simulink model "fullDiveHarness"  (R2026a)
settings: Solver=ode23t  StopTime=3900  MaxStep=0.1  RelTol=1e-4
libraries: simulink x2
settings Model: Creator=grouleau  LastModifiedBy=grouleau

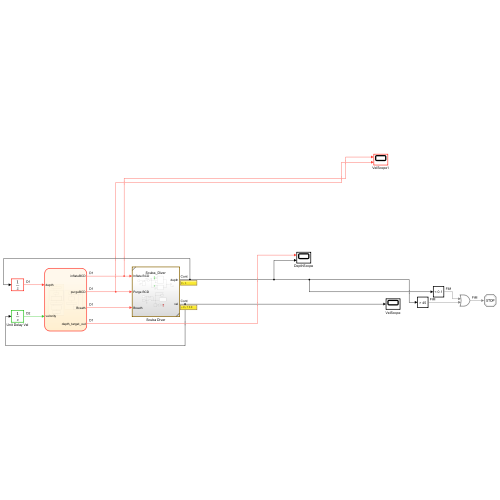
[thumbnail: Simulink's stored preview of the top-level diagram]
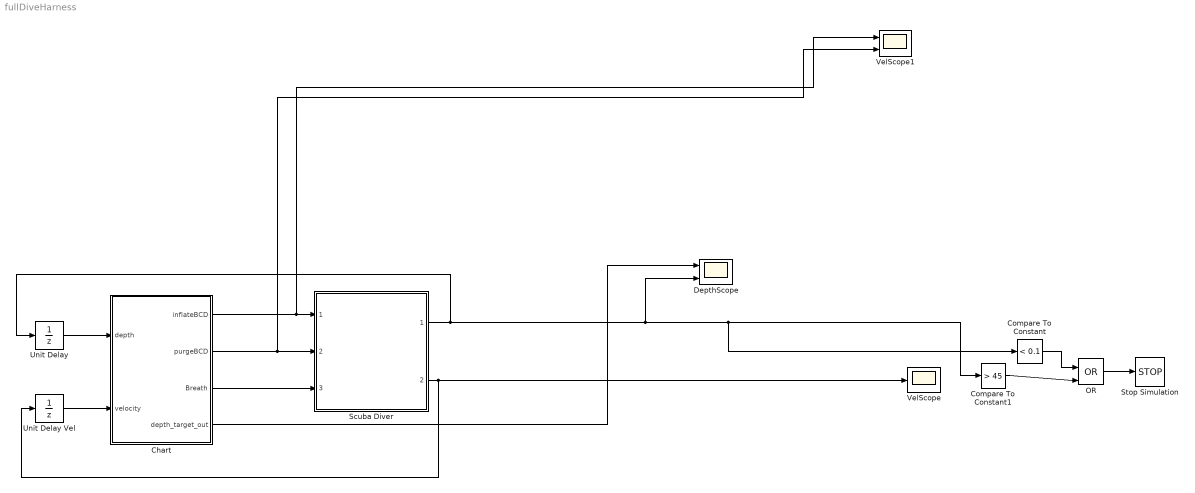
== system fullDiveHarness ==
  Chart : Stateflow chart  TreatAsAtomicUnit=on
  Compare To Constant : simulink/Logic and Bit Operations/Compare To Constant  relop=<  const=0.1  OutDataTypeStr=boolean
  Compare To Constant1 : simulink/Logic and Bit Operations/Compare To Constant  relop=>  const=45  OutDataTypeStr=boolean
  DepthScope : Scope  NumInputPorts=2
      settings: ActiveDisplayYMinimum=-1.029122167100595  ActiveDisplayYMaximum=9.2620995039053575
  OR : Logic  Operator=OR  IconShape=distinctive  AllPortsSameDT=off  OutDataTypeStr=boolean
  Scuba Diver : Subsystem  ReferencedSubsystem=Scuba_Diver
  Stop Simulation : Stop
  Unit Delay : UnitDelay  InitialCondition=20  SampleTime=0.01
  Unit Delay Vel : UnitDelay  SampleTime=0.1
  VelScope : Scope
      settings: ActiveDisplayYMinimum=-0.68143414282353132  ActiveDisplayYMaximum=0.60845700128408264
  VelScope1 : Scope  NumInputPorts=2
      settings: ActiveDisplayYMinimum=-1  ActiveDisplayYMaximum=1
  wires:
  Unit Delay Vel/1 -> Chart/2(velocity)
  Scuba Diver/1 -> DepthScope/2, Compare To Constant1/1, Compare To Constant/1, Unit Delay/1
  Compare To Constant1/1 -> OR/2
  OR/1 -> Stop Simulation/1
  Compare To Constant/1 -> OR/1
  Chart/3(Breath) -> Scuba Diver/3
  Scuba Diver/2 -> VelScope/1, Unit Delay Vel/1
  Chart/2(purgeBCD) -> VelScope1/2, Scuba Diver/2
  Chart/1(inflateBCD) -> VelScope1/1, Scuba Diver/1
  Unit Delay/1 -> Chart/1(depth)
  Chart/4(depth_target_out) -> DepthScope/1

== stateflow chart fullDiveHarness/Chart ==
  state BCD_Supervisor [parallel]
    en:
    depth_target = 0.0;
    du:
    depth_target_out = depth_target;
    settings: executionOrder=1
    state DESCENT
      du:
      depth_target = min(ctrl_bottom_depth, ctrl_descent_rate * elapsed(sec));
      if velocity > ctrl_max_descent_rate
      inflateBCD = ctrl_K_brake * (velocity - ctrl_max_descent_rate);
      else
      inflateBCD = 0.0;
      end
      purgeBCD = 0.0;
    state BOTTOM_HOLD
      state NEUTRAL_BURST
        en:
        inflateBCD = 1.0;
        purgeBCD = 0.0;
        depth_target = ctrl_bottom_depth;
      state HOLD
        en:
        inflateBCD = 0.0;
        purgeBCD = 0.0;
        du:
        depth_target = ctrl_bottom_depth;
        if ctrl_bottom_depth - depth > ctrl_bcd_deadband
        purgeBCD = ctrl_K_p * ((ctrl_bottom_depth - depth) - ctrl_bcd_deadband);
        inflateBCD = 0.0;
        elseif ctrl_bottom_depth - depth < -ctrl_bcd_deadband
        inflateBCD = ctrl_K_p * (abs(ctrl_bottom_depth - depth) - ctrl_bcd_deadband);
        purgeBCD = 0.0;
        else
        inflateBCD = 0.0;
        purgeBCD = 0.0;
        end
      (default) -> NEUTRAL_BURST
      NEUTRAL_BURST -> HOLD : [elapsed(sec) >= ctrl_neutral_burst_duration]
    state ASCEND
      du:
      depth_target = max(ctrl_safety_depth, ctrl_bottom_depth - ctrl_ascent_rate * elapsed(sec));
      purgeBCD = ctrl_K_ascent * max(0.0, -velocity);
      if -velocity > ctrl_max_ascent_rate
      purgeBCD = 1.0;
      end
      inflateBCD = 0.0;
    state SAFETY_STOP
      du:
      depth_target = ctrl_safety_depth;
      if ctrl_safety_depth - depth > ctrl_bcd_deadband
      purgeBCD = ctrl_K_p * ((ctrl_safety_depth - depth) - ctrl_bcd_deadband);
      inflateBCD = 0.0;
      elseif ctrl_safety_depth - depth < -ctrl_bcd_deadband
      inflateBCD = ctrl_K_p * (abs(ctrl_safety_depth - depth) - ctrl_bcd_deadband);
      purgeBCD = 0.0;
      else
      inflateBCD = 0.0;
      purgeBCD = 0.0;
      end
    state FINAL_ASCENT
      du:
      depth_target = max(1.0, ctrl_safety_depth - 0.0267 * elapsed(sec));
      purgeBCD = ctrl_K_ascent * max(0.0, -velocity);
      if -velocity > ctrl_max_ascent_rate
      purgeBCD = 1.0;
      end
      inflateBCD = 0.0;
    state SURFACED
      du:
      depth_target = 1.0;
      inflateBCD = 1.0;
      purgeBCD = 0.0;
    (default) -> DESCENT
    DESCENT -> BOTTOM_HOLD : [depth_target >= ctrl_bottom_depth]
    BOTTOM_HOLD -> ASCEND : [elapsed(sec) >= ctrl_bottom_duration]
    ASCEND -> SAFETY_STOP : [depth_target <= ctrl_safety_depth]
    SAFETY_STOP -> FINAL_ASCENT : [elapsed(sec) >= ctrl_safety_duration]
    FINAL_ASCENT -> SURFACED : [depth_target <= 1.0]
  state Breathing_Controller [parallel]
    en:
    bias = 0.0;
    bias_input = 0.0;
    du:
    bias_input = (depth - depth_target) + bc_K_vel * velocity;
    if bias_input < -bc_saturation
    bias = -1.0;
    elseif bias_input > bc_saturation
    bias = 1.0;
    elseif (bias_input > -bc_deadzone) && (bias_input < bc_deadzone)
    bias = 0.0;
    elseif bias_input >= bc_deadzone
    bias = (bias_input - bc_deadzone) / (bc_saturation - bc_deadzone);
    else
    bias = (bias_input + bc_deadzone) / (bc_saturation - bc_deadzone);
    end
    settings: executionOrder=2
    state Inhale
      en:
      if bias >= 0.0
      t_inh = bc_t_inh_0 * (1.0 + bc_duty_shift_inh * bias);
      else
      t_inh = bc_t_inh_0 * (1.0 + 0.1 * bias);
      end
      A_inhale = bc_A_base * (1.0 + bc_amplitude_gain * bias) * (1.0 + depth / 40.0);
      Breath = -A_inhale;
    state Inhale_Hold
      en:
      if bias >= 0.0
      t_ihld = bc_t_ihld_0 + bc_hold_shift_max * bias;
      else
      t_ihld = bc_t_ihld_0 + 0.9 * bias;
      if t_ihld < 0.1
      t_ihld = 0.1;
      end
      end
      Breath = 0.0;
    state Exhale
      en:
      if bias >= 0.0
      t_exh = bc_t_exh_0 * (1.0 - 0.1 * bias);
      else
      t_exh = bc_t_exh_0 * (1.0 - bc_duty_shift_exh * bias);
      end
      A_exhale = bc_A_base * (1.0 - bc_amplitude_gain * bias) * (1.0 + depth / 40.0);
      Breath = A_exhale;
    state Exhale_Hold
      en:
      if bias >= 0.0
      t_ehld = bc_t_ehld_0 - 0.9 * bias;
      if t_ehld < 0.1
      t_ehld = 0.1;
      end
      else
      t_ehld = bc_t_ehld_0 - bc_hold_shift_max * bias;
      end
      Breath = 0.0;
    (default) -> Inhale
    Inhale -> Inhale_Hold : after(t_inh, sec)
    Exhale_Hold -> Inhale : after(t_ehld, sec)
    Inhale_Hold -> Exhale : after(t_ihld, sec)
    Exhale -> Exhale_Hold : after(t_exh, sec)
  data: inflateBCD output double =0; purgeBCD output double =0; Breath output =0; depth input; velocity input double; bias_input local double; bias local double; t_inh local double; t_ihld local double; t_exh local double; t_ehld local double; A_inhale local double; A_exhale local double; ctrl_bottom_depth parameter; ctrl_descent_rate parameter; ctrl_max_descent_rate parameter; ctrl_K_brake parameter; ctrl_bottom_duration parameter; ctrl_safety_depth parameter; ctrl_bcd_deadband parameter; ctrl_K_p parameter; ctrl_ascent_rate parameter; ctrl_K_ascent parameter; ctrl_max_ascent_rate parameter; ctrl_safety_duration parameter; ctrl_neutral_burst_duration parameter; bc_t_inh_0 parameter; bc_duty_shift_inh parameter; bc_A_base parameter; bc_amplitude_gain parameter; bc_t_ihld_0 parameter; bc_hold_shift_max parameter; bc_t_exh_0 parameter; bc_duty_shift_exh parameter; bc_t_ehld_0 parameter; bc_K_vel parameter; bc_saturation parameter; bc_deadzone parameter; depth_target local double; depth_target_out output double
